simulink model "closed_loop_with_control"  (R2017b)
settings: Solver=VariableStepAuto  StartTime=0.0  StopTime=10.0  RelTol=1e-3
settings Model: Creator=nadav  LastModifiedBy=nadav

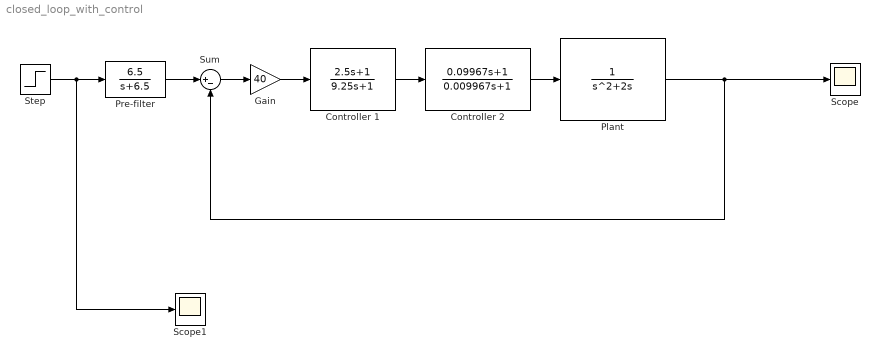
== system closed_loop_with_control ==
  "Controller 1 " : TransferFcn  Numerator=[2.5 1]  Denominator=[9.25 1]
  "Controller 2 " : TransferFcn  Numerator=[0.09967 1]  Denominator=[0.009967 1]
  Gain : Gain  Gain=40
  "Plant " : TransferFcn  Denominator=[1 2 0]
  Pre-filter : TransferFcn  Numerator=[6.5]  Denominator=[1 6.5]
  Scope : Scope
  Scope1 : Scope
  Step : Step  Time=0  SampleTime=0
  Sum : Sum  Inputs=|+-
  wires:
  Step/1 -> Scope1/1, Pre-filter/1
  Gain/1 -> "Controller 1 "/1
  "Plant "/1 -> Sum/2, Scope/1
  Sum/1 -> Gain/1
  "Controller 1 "/1 -> "Controller 2 "/1
  "Controller 2 "/1 -> "Plant "/1
  Pre-filter/1 -> Sum/1
